simulink model "PeakDetect3"  (R2018b)
settings: Solver=FixedStepAuto  StartTime=0  StopTime=500*(15e-9)  FixedStep=15e-9  RelTol=1e-3
libraries: simulink x35, hdlsllib x34
(part 2 of 4)

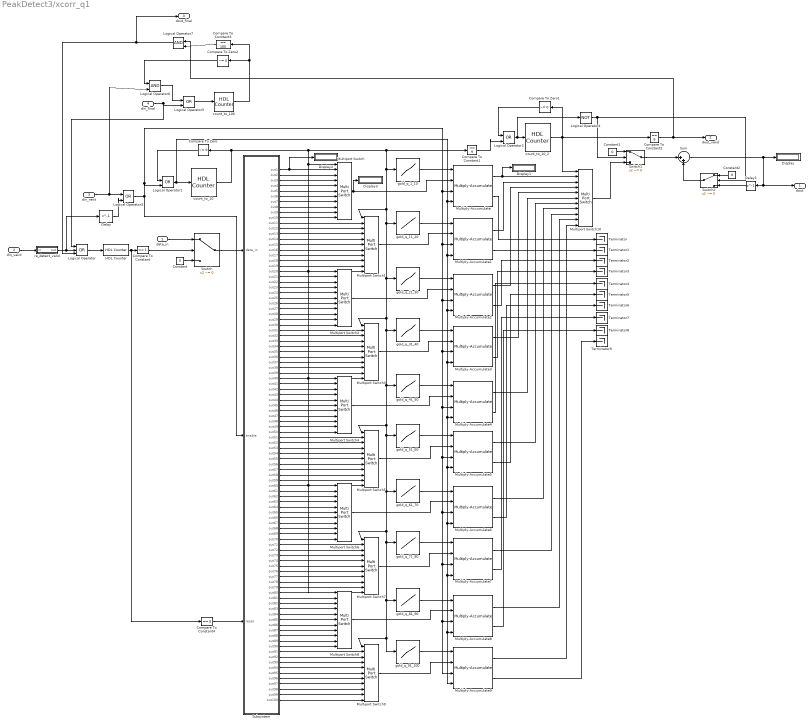
== system PeakDetect3/xcorr_q1 ==
  data_in : Inport  OutDataTypeStr=fixdt(1,16,15)
  din_valid : Inport  Port=2
  din_next : Inport  Port=3
  din_final : Inport  Port=4
  Compare To Constant : simulink/Logic and Bit Operations/Compare To Constant  relop===  const=1  OutDataTypeStr=boolean
  Compare To Constant1 : simulink/Logic and Bit Operations/Compare To Constant  relop===  const=9  OutDataTypeStr=boolean
  Compare To Constant2 : simulink/Logic and Bit Operations/Compare To Constant  relop===  const=9  OutDataTypeStr=boolean
  Compare To Constant3 : simulink/Logic and Bit Operations/Compare To Constant  relop===  const=100  OutDataTypeStr=boolean
  Compare To Constant4 : simulink/Logic and Bit Operations/Compare To Constant  relop===  const=0  OutDataTypeStr=boolean
  Compare To Zero : simulink/Logic and Bit Operations/Compare To Zero  relop=~=  OutDataTypeStr=boolean
  Compare To Zero1 : simulink/Logic and Bit Operations/Compare To Zero  relop=~=  OutDataTypeStr=boolean
  Compare To Zero2 : simulink/Logic and Bit Operations/Compare To Zero  relop=~=  OutDataTypeStr=boolean
  Constant : Constant  Value=0  OutDataTypeStr=fixdt(1,16,15)  SampleTime=-1
  Constant1 : Constant  Value=0  OutDataTypeStr=Inherit: Inherit via back propagation  SampleTime=-1
  Constant2 : Constant  Value=0  OutDataTypeStr=Inherit: Inherit via back propagation  SampleTime=-1
  Delay : Delay  DelayLength=1
  Delay1 : Delay  DelayLength=1
  Display{,1..3} (4 alike) : Display
  HDL Counter : hdlsllib/Sources/HDL Counter  CountType=Count limited  CountInit=0  CountStep=1  CountMax=2  CountFromType=Initial value  CountFrom=0  CountResetPort=off  CountLoadPort=off  CountEnbPort=on  CountDirPort=off  CountDataType=Unsigned  CountWordLen=8  CountFracLen=0  CountSampTime=1
      settings: SourceProductBaseCode=HD
  Logical Operator : Logic  Operator=OR  Inputs=3  IconShape=distinctive  AllPortsSameDT=off  OutDataTypeStr=boolean
  Logical Operator{1..3,5} (4 alike) : Logic  Operator=OR  IconShape=distinctive  AllPortsSameDT=off  OutDataTypeStr=boolean
  Logical Operator4 : Logic  Operator=NOT  IconShape=distinctive  AllPortsSameDT=off  OutDataTypeStr=boolean
  Logical Operator6 : Logic  IconShape=distinctive  AllPortsSameDT=off  OutDataTypeStr=boolean
  Logical Operator7 : Logic  IconShape=distinctive  AllPortsSameDT=off  OutDataTypeStr=boolean
  Multiply-Accumulate{,1..9} (10 alike) : hdlsllib/HDL Operations/Multiply-Accumulate  opMode=Streaming - using Start and End ports  initValueSetting=Dialog  initValue=0  initValueSetting2=Dialog  initValue2=0  initValueSetting3=Dialog  initValue3=0  num_samples=2  RndMeth2=Floor  RndMeth3=Floor  datatype2=fixdt(1,32,16)  datatype3=Inherit: Inherit via back propagation  validOut=on  endInandOut=off  startOut=off  countOut=on  dim=-1  DoSatur=off  parallel=off
      settings: SourceProductName=HDL Coder  SourceProductBaseCode=HD
  Multiport Switch{,1..9} (10 alike) : MultiPortSwitch  DataPortOrder=Zero-based contiguous  Inputs=10  zeroidx=on  OutDataTypeStr=fixdt(1,16,15)
  Multiport Switch10 : MultiPortSwitch  DataPortOrder=Zero-based contiguous  Inputs=10  zeroidx=on  OutDataTypeStr=fixdt(1,32,16)
  Subsystem : Subsystem
  Sum : Sum  Inputs=|++  OutDataTypeStr=Inherit: Inherit via back propagation
  Switch : Switch  Criteria=u2 ~= 0  OutDataTypeStr=Inherit: Inherit via back propagation
  Switch1 : Switch  Criteria=u2 ~= 0  OutDataTypeStr=Inherit: Inherit via back propagation
  Switch2 : Switch  Criteria=u2 ~= 0  OutDataTypeStr=Inherit: Inherit via back propagation
  Terminator{,1..9} (10 alike) : Terminator
  count_to_10 : hdlsllib/Sources/HDL Counter  CountType=Count limited  CountInit=0  CountStep=1  CountMax=9  CountFromType=Initial value  CountFrom=0  CountResetPort=off  CountLoadPort=off  CountEnbPort=on  CountDirPort=off  CountDataType=Unsigned  CountWordLen=4  CountFracLen=0  CountSampTime=1
      settings: SourceProductBaseCode=HD
  count_to_100 : hdlsllib/Sources/HDL Counter  CountType=Count limited  CountInit=0  CountStep=1  CountMax=100  CountFromType=Initial value  CountFrom=0  CountResetPort=off  CountLoadPort=off  CountEnbPort=on  CountDirPort=off  CountDataType=Unsigned  CountWordLen=8  CountFracLen=0  CountSampTime=1
      settings: SourceProductBaseCode=HD
  count_to_10_2 : hdlsllib/Sources/HDL Counter  CountType=Count limited  CountInit=0  CountStep=1  CountMax=9  CountFromType=Initial value  CountFrom=0  CountResetPort=off  CountLoadPort=off  CountEnbPort=on  CountDirPort=off  CountDataType=Unsigned  CountWordLen=4  CountFracLen=0  CountSampTime=1
      settings: SourceProductBaseCode=HD
  gold_q_11_20 : Lookup_n-D  NumberOfTableDimensions=1  LookupTableObject=''  BreakpointsForDimension1=uint8([0,1,2,3,4,5,6,7,8,9])  BreakpointsForDimension1FirstPoint=10  BreakpointsForDimension2FirstPoint=10  BreakpointsForDimension1Spacing=12  BreakpointsForDimension2Spacing=12  IndexSearchMethod=Evenly spaced points  Table=|  TableDataTypeStr=fixdt(1,16,15)  InterpMethod=Flat  DiagnosticForOutOfRangeInput=Error  InternalRulePriority=Speed  OutDataTypeStr=fixdt(1,16,15)  RndMeth=Simplest  InputSameDT=on
      | -1*[0.236906374990369
      | 0.265062589296935
      | 0.290853922757751
      | 0.306866645010829
      | 0.306877356493505
      | 0.282583044796408
      | 0.237895318583737
      | 0.179451570247324
      | 0.106711739895776
      | 0.0250742736874029]
  gold_q_1_10 : Lookup_n-D  NumberOfTableDimensions=1  LookupTableObject=''  BreakpointsForDimension1=uint8([0,1,2,3,4,5,6,7,8,9])  BreakpointsForDimension1FirstPoint=10  BreakpointsForDimension2FirstPoint=10  BreakpointsForDimension1Spacing=12  BreakpointsForDimension2Spacing=12  IndexSearchMethod=Evenly spaced points  Table=|  TableDataTypeStr=fixdt(1,16,15)  InterpMethod=Flat  DiagnosticForOutOfRangeInput=Error  InternalRulePriority=Speed  OutDataTypeStr=fixdt(1,16,15)  RndMeth=Simplest  InputSameDT=on
      | -1*[0.357169275362262
      | 0.373691122276015
      | 0.363136475782144
      | 0.332586509539436
      | 0.291374087870011
      | 0.249422279627694
      | 0.215579045674242
      | 0.200455944131647
      | 0.201796906991478
      | 0.213779029408702]
  gold_q_21_30 : Lookup_n-D  NumberOfTableDimensions=1  LookupTableObject=''  BreakpointsForDimension1=uint8([0,1,2,3,4,5,6,7,8,9])  BreakpointsForDimension1FirstPoint=10  BreakpointsForDimension2FirstPoint=10  BreakpointsForDimension1Spacing=12  BreakpointsForDimension2Spacing=12  IndexSearchMethod=Evenly spaced points  Table=|  TableDataTypeStr=fixdt(1,16,15)  InterpMethod=Flat  DiagnosticForOutOfRangeInput=Error  InternalRulePriority=Speed  OutDataTypeStr=fixdt(1,16,15)  RndMeth=Simplest  InputSameDT=on
      | -1*[-0.0591515848508664
      | -0.139598314313151
      | -0.210629837752387
      | -0.263713716480122
      | -0.301489962058033
      | -0.328238114626508
      | -0.340130412877520
      | -0.338689881672749
      | -0.326243180584237
      | -0.305614110780615]
  gold_q_31_40 : Lookup_n-D  NumberOfTableDimensions=1  LookupTableObject=''  BreakpointsForDimension1=uint8([0,1,2,3,4,5,6,7,8,9])  BreakpointsForDimension1FirstPoint=10  BreakpointsForDimension2FirstPoint=10  BreakpointsForDimension1Spacing=12  BreakpointsForDimension2Spacing=12  IndexSearchMethod=Evenly spaced points  Table=|  TableDataTypeStr=fixdt(1,16,15)  InterpMethod=Flat  DiagnosticForOutOfRangeInput=Error  InternalRulePriority=Speed  OutDataTypeStr=fixdt(1,16,15)  RndMeth=Simplest  InputSameDT=on
      | -1*[-0.279858098355888
      | -0.247814863771713
      | -0.225446174923891
      | -0.202743193363060
      | -0.186527042991191
      | -0.178781266249413
      | -0.180711431323688
      | -0.192575241083779
      | -0.213551675353351
      | -0.245925394077466]
  gold_q_41_50 : Lookup_n-D  NumberOfTableDimensions=1  LookupTableObject=''  BreakpointsForDimension1=uint8([0,1,2,3,4,5,6,7,8,9])  BreakpointsForDimension1FirstPoint=10  BreakpointsForDimension2FirstPoint=10  BreakpointsForDimension1Spacing=12  BreakpointsForDimension2Spacing=12  IndexSearchMethod=Evenly spaced points  Table=|  TableDataTypeStr=fixdt(1,16,15)  InterpMethod=Flat  DiagnosticForOutOfRangeInput=Error  InternalRulePriority=Speed  OutDataTypeStr=fixdt(1,16,15)  RndMeth=Simplest  InputSameDT=on
      | -1*[-0.273649789754997
      | -0.305507933389466
      | -0.332526349511340
      | -0.349961882407133
      | -0.353614169955030
      | -0.340366684130075
      | -0.308641627170326
      | -0.254460428744123
      | -0.185247665828561
      | -0.110080691949015]
  gold_q_51_60 : Lookup_n-D  NumberOfTableDimensions=1  LookupTableObject=''  BreakpointsForDimension1=uint8([0,1,2,3,4,5,6,7,8,9])  BreakpointsForDimension1FirstPoint=10  BreakpointsForDimension2FirstPoint=10  BreakpointsForDimension1Spacing=12  BreakpointsForDimension2Spacing=12  IndexSearchMethod=Evenly spaced points  Table=|  TableDataTypeStr=fixdt(1,16,15)  InterpMethod=Flat  DiagnosticForOutOfRangeInput=Error  InternalRulePriority=Speed  OutDataTypeStr=fixdt(1,16,15)  RndMeth=Simplest  InputSameDT=on
      | -1*[-0.0297558495000079
      | 0.0499350486257353
      | 0.122950591883728
      | 0.183532283875116
      | 0.226715241693549
      | 0.244522518247979
      | 0.247772413924009
      | 0.223279362418140
      | 0.176793915855740
      | 0.111355596734925]
  gold_q_61_70 : Lookup_n-D  NumberOfTableDimensions=1  LookupTableObject=''  BreakpointsForDimension1=uint8([0,1,2,3,4,5,6,7,8,9])  BreakpointsForDimension1FirstPoint=10  BreakpointsForDimension2FirstPoint=10  BreakpointsForDimension1Spacing=12  BreakpointsForDimension2Spacing=12  IndexSearchMethod=Evenly spaced points  Table=|  TableDataTypeStr=fixdt(1,16,15)  InterpMethod=Flat  DiagnosticForOutOfRangeInput=Error  InternalRulePriority=Speed  OutDataTypeStr=fixdt(1,16,15)  RndMeth=Simplest  InputSameDT=on
      | -1*[0.0312880626224120
      | -0.0580988665112754
      | -0.150830519884918
      | -0.236354458852815
      | -0.321361371110983
      | -0.387151947785857
      | -0.432910784333285
      | -0.454553321854592
      | -0.449340647995131
      | -0.416266380216616]
  gold_q_71_80 : Lookup_n-D  NumberOfTableDimensions=1  LookupTableObject=''  BreakpointsForDimension1=uint8([0,1,2,3,4,5,6,7,8,9])  BreakpointsForDimension1FirstPoint=10  BreakpointsForDimension2FirstPoint=10  BreakpointsForDimension1Spacing=12  BreakpointsForDimension2Spacing=12  IndexSearchMethod=Evenly spaced points  Table=|  TableDataTypeStr=fixdt(1,16,15)  InterpMethod=Flat  DiagnosticForOutOfRangeInput=Error  InternalRulePriority=Speed  OutDataTypeStr=fixdt(1,16,15)  RndMeth=Simplest  InputSameDT=on
      | -1*[-0.356405677154333
      | -0.268905527196357
      | -0.172503144328213
      | -0.0623088722264564
      | 0.0478292512438748
      | 0.147701871156711
      | 0.227579808283800
      | 0.279365016179912
      | 0.297653875710056
      | 0.276310228166542]
  gold_q_81_90 : Lookup_n-D  NumberOfTableDimensions=1  LookupTableObject=''  BreakpointsForDimension1=uint8([0,1,2,3,4,5,6,7,8,9])  BreakpointsForDimension1FirstPoint=10  BreakpointsForDimension2FirstPoint=10  BreakpointsForDimension1Spacing=12  BreakpointsForDimension2Spacing=12  IndexSearchMethod=Evenly spaced points  Table=|  TableDataTypeStr=fixdt(1,16,15)  InterpMethod=Flat  DiagnosticForOutOfRangeInput=Error  InternalRulePriority=Speed  OutDataTypeStr=fixdt(1,16,15)  RndMeth=Simplest  InputSameDT=on
      | -1*[0.222595237130309
      | 0.147485843722747
      | 0.0555170073150737
      | -0.0424496465550990
      | -0.134707118174198
      | -0.210100315272752
      | -0.259403813850479
      | -0.272248751146779
      | -0.259403813850479
      | -0.210100315272752]
  gold_q_91_100 : Lookup_n-D  NumberOfTableDimensions=1  LookupTableObject=''  BreakpointsForDimension1=uint8([0,1,2,3,4,5,6,7,8,9])  BreakpointsForDimension1FirstPoint=10  BreakpointsForDimension2FirstPoint=10  BreakpointsForDimension1Spacing=12  BreakpointsForDimension2Spacing=12  IndexSearchMethod=Evenly spaced points  Table=|  TableDataTypeStr=fixdt(1,16,15)  InterpMethod=Flat  DiagnosticForOutOfRangeInput=Error  InternalRulePriority=Speed  OutDataTypeStr=fixdt(1,16,15)  RndMeth=Simplest  InputSameDT=on
      | -1*[-0.134707118174198
      | -0.0424496465550989
      | 0.0555170073150737
      | 0.147485843722747
      | 0.222595237130309
      | 0.267820298855522
      | 0.290378842162360
      | 0.275261187855880
      | 0.228204197191429
      | 0.153805243290024]
  re_detect_valid : Subsystem
  dout : Outport  OutDataTypeStr=fixdt(1,32,16)
  dout_valid : Outport  Port=2
  dout_final : Outport  Port=3
  wires:
  Subsystem/63(out63) -> Multiport Switch6/4
  Subsystem/83(out83) -> Multiport Switch8/4
  Subsystem/87(out87) -> Multiport Switch8/8
  Subsystem/57(out57) -> Multiport Switch5/8
  count_to_10/1 -> Compare To Zero/1, Multiport Switch8/1, Multiport Switch6/1, Multiport Switch4/1, Multiport Switch2/1, Multiport Switch/1, gold_q_11_20/1, gold_q_21_30/1, gold_q_31_40/1, gold_q_41_50/1, gold_q_51_60/1, gold_q_61_70/1, gold_q_71_80/1, gold_q_81_90/1, gold_q_91_100/1, Multiport Switch9/1, Multiport Switch7/1, Multiport Switch5/1, Multiport Switch3/1, Multiport Switch1/1, gold_q_1_10/1, Compare To Constant1/1
  Subsystem/97(out97) -> Multiport Switch9/8
  Multiply-Accumulate4/1 -> Multiport Switch10/6
  Subsystem/65(out65) -> Multiport Switch6/6
  Subsystem/99(out99) -> Multiport Switch9/10
  Subsystem/73(out73) -> Multiport Switch7/4
  Subsystem/49(out49) -> Multiport Switch4/10
  Multiply-Accumulate/2 -> Terminator/1
  din_final/1 -> Logical Operator/1, Logical Operator5/2
  count_to_10_2/1 -> Compare To Constant2/1, Multiport Switch10/1, Compare To Zero1/1
  Multiport Switch8/1 -> Multiply-Accumulate8/2
  Compare To Constant2/1 -> dout_valid/1, Logical Operator7/1
  Subsystem/61(out61) -> Multiport Switch6/2
  Subsystem/28(out28) -> Multiport Switch2/9
  Subsystem/1(out1) -> Display2/1, Multiport Switch/2
  Multiply-Accumulate6/1 -> Multiport Switch10/8
  Subsystem/100(out100) -> Multiport Switch9/11
  Logical Operator/1 -> HDL Counter/1
  din_valid/1 -> re_detect_valid/1(in)
  Subsystem/68(out68) -> Multiport Switch6/9
  Subsystem/56(out56) -> Multiport Switch5/7
  Subsystem/13(out13) -> Multiport Switch1/4
  Subsystem/67(out67) -> Multiport Switch6/8
  Subsystem/66(out66) -> Multiport Switch6/7
  Logical Operator2/1 -> Logical Operator4/1, count_to_10_2/1
  Constant/1 -> Switch/3
  Compare To Zero/1 -> Logical Operator1/1
  Subsystem/89(out89) -> Multiport Switch8/10
  Multiport Switch5/1 -> Multiply-Accumulate5/2
  Subsystem/29(out29) -> Multiport Switch2/10
  Compare To Constant/1 -> Switch/2
  gold_q_91_100/1 -> Multiply-Accumulate9/1
  Subsystem/52(out52) -> Multiport Switch5/3
  re_detect_valid/1(out) -> Delay/1, Logical Operator/2
  Logical Operator1/1 -> count_to_10/1, Multiply-Accumulate2/4, Multiply-Accumulate9/4, Multiply-Accumulate8/4, Multiply-Accumulate7/4, Multiply-Accumulate6/4, Multiply-Accumulate5/4, Multiply-Accumulate4/4, Multiply-Accumulate3/4, Multiply-Accumulate1/4, Multiply-Accumulate/4
  Subsystem/76(out76) -> Multiport Switch7/7
  Sum/1 -> dout/1, Delay1/1, Display/1
  Logical Operator3/1 -> Subsystem/2(enable), Multiply-Accumulate9/3, Multiply-Accumulate8/3, Multiply-Accumulate7/3, Multiply-Accumulate6/3, Multiply-Accumulate5/3, Multiply-Accumulate4/3, Multiply-Accumulate3/3, Multiply-Accumulate2/3, Multiply-Accumulate1/3, Multiply-Accumulate/3, Logical Operator1/2
  Subsystem/2(out2) -> Multiport Switch/3
  Subsystem/88(out88) -> Multiport Switch8/9
  Subsystem/64(out64) -> Multiport Switch6/5
  Subsystem/41(out41) -> Multiport Switch4/2
  Multiply-Accumulate9/2 -> Terminator9/1
  din_next/1 -> Logical Operator6/2, Logical Operator3/1
  Subsystem/11(out11) -> Multiport Switch1/2
  Subsystem/96(out96) -> Multiport Switch9/7
  Switch1/1 -> Sum/1
  Subsystem/80(out80) -> Multiport Switch7/11
  Subsystem/54(out54) -> Multiport Switch5/5
  Subsystem/82(out82) -> Multiport Switch8/3
  Multiply-Accumulate4/2 -> Terminator4/1
  Subsystem/6(out6) -> Multiport Switch/7
  Subsystem/45(out45) -> Multiport Switch4/6
  Multiport Switch4/1 -> Multiply-Accumulate4/2
  Logical Operator4/1 -> Switch1/2, Switch2/2
  Subsystem/58(out58) -> Multiport Switch5/9
  Subsystem/81(out81) -> Multiport Switch8/2
  Subsystem/44(out44) -> Multiport Switch4/5
  Subsystem/86(out86) -> Multiport Switch8/7
  Subsystem/85(out85) -> Multiport Switch8/6
  Logical Operator5/1 -> count_to_100/1
  Multiport Switch/1 -> Multiply-Accumulate/2, Display3/1
  Subsystem/27(out27) -> Multiport Switch2/8
  gold_q_31_40/1 -> Multiply-Accumulate3/1
  Subsystem/93(out93) -> Multiport Switch9/4
  Compare To Zero1/1 -> Logical Operator2/1
  Subsystem/39(out39) -> Multiport Switch3/10
  Subsystem/84(out84) -> Multiport Switch8/5
  Subsystem/70(out70) -> Multiport Switch6/11
  Subsystem/77(out77) -> Multiport Switch7/8
  Subsystem/62(out62) -> Multiport Switch6/3
  Subsystem/95(out95) -> Multiport Switch9/6
  gold_q_1_10/1 -> Multiply-Accumulate/1
  Compare To Zero2/1 -> Logical Operator6/1
  Multiply-Accumulate1/1 -> Multiport Switch10/3
  Subsystem/47(out47) -> Multiport Switch4/8
  Multiply-Accumulate3/2 -> Terminator3/1
  Subsystem/22(out22) -> Multiport Switch2/3
  Subsystem/92(out92) -> Multiport Switch9/3
  count_to_100/1 -> Compare To Constant3/1, Compare To Zero2/1
  Multiport Switch3/1 -> Multiply-Accumulate3/2
  Subsystem/59(out59) -> Multiport Switch5/10
  Subsystem/9(out9) -> Multiport Switch/10
  Subsystem/5(out5) -> Multiport Switch/6
  gold_q_11_20/1 -> Multiply-Accumulate1/1
  data_in/1 -> Switch/1
  Subsystem/90(out90) -> Multiport Switch8/11
  Subsystem/10(out10) -> Multiport Switch/11
  Subsystem/75(out75) -> Multiport Switch7/6
  Subsystem/18(out18) -> Multiport Switch1/9
  Subsystem/12(out12) -> Multiport Switch1/3
  Subsystem/25(out25) -> Multiport Switch2/6
  Subsystem/43(out43) -> Multiport Switch4/4
  Subsystem/72(out72) -> Multiport Switch7/3
  Subsystem/30(out30) -> Multiport Switch2/11
  Subsystem/8(out8) -> Multiport Switch/9
  Subsystem/60(out60) -> Multiport Switch5/11
  HDL Counter/1 -> Compare To Constant4/1, Compare To Constant/1
  Multiply-Accumulate8/2 -> Terminator8/1
  Subsystem/17(out17) -> Multiport Switch1/8
  Multiply-Accumulate9/1 -> Multiport Switch10/11
  Subsystem/26(out26) -> Multiport Switch2/7
  Subsystem/35(out35) -> Multiport Switch3/6
  Subsystem/24(out24) -> Multiport Switch2/5
  Subsystem/20(out20) -> Multiport Switch1/11
  Subsystem/71(out71) -> Multiport Switch7/2
  Subsystem/78(out78) -> Multiport Switch7/9
  Multiport Switch9/1 -> Multiply-Accumulate9/2
  Subsystem/7(out7) -> Multiport Switch/8
  Subsystem/3(out3) -> Multiport Switch/4
  Subsystem/79(out79) -> Multiport Switch7/10
  Multiport Switch10/1 -> Switch1/3
  Subsystem/15(out15) -> Multiport Switch1/6
  Subsystem/14(out14) -> Multiport Switch1/5
  Multiply-Accumulate/1 -> Display1/1, Multiport Switch10/2
  Subsystem/42(out42) -> Multiport Switch4/3
  Subsystem/16(out16) -> Multiport Switch1/7
  Logical Operator6/1 -> Logical Operator5/1
  Logical Operator7/1 -> dout_final/1, Logical Operator/3
  Subsystem/53(out53) -> Multiport Switch5/4
  Subsystem/37(out37) -> Multiport Switch3/8
  Subsystem/55(out55) -> Multiport Switch5/6
  Subsystem/48(out48) -> Multiport Switch4/9
  Subsystem/4(out4) -> Multiport Switch/5
  Subsystem/50(out50) -> Multiport Switch4/11
  Subsystem/40(out40) -> Multiport Switch3/11
  Switch/1 -> Subsystem/1(data_in)
  Subsystem/19(out19) -> Multiport Switch1/10
  Subsystem/38(out38) -> Multiport Switch3/9
  Subsystem/33(out33) -> Multiport Switch3/4
  Subsystem/46(out46) -> Multiport Switch4/7
  Subsystem/31(out31) -> Multiport Switch3/2
  Subsystem/69(out69) -> Multiport Switch6/10
  Subsystem/94(out94) -> Multiport Switch9/5
  gold_q_71_80/1 -> Multiply-Accumulate7/1
  Subsystem/32(out32) -> Multiport Switch3/3
  Multiply-Accumulate3/1 -> Multiport Switch10/5
  Subsystem/23(out23) -> Multiport Switch2/4
  Multiply-Accumulate2/1 -> Multiport Switch10/4
  Multiport Switch6/1 -> Multiply-Accumulate6/2
  Constant1/1 -> Switch1/1
  Multiply-Accumulate6/2 -> Terminator6/1
  Compare To Constant1/1 -> Logical Operator2/2
  Constant2/1 -> Switch2/1
  Compare To Constant3/1 -> Logical Operator7/2
  gold_q_41_50/1 -> Multiply-Accumulate4/1
  gold_q_21_30/1 -> Multiply-Accumulate2/1
  Multiport Switch2/1 -> Multiply-Accumulate2/2
  Subsystem/21(out21) -> Multiport Switch2/2
  gold_q_61_70/1 -> Multiply-Accumulate6/1
  gold_q_51_60/1 -> Multiply-Accumulate5/1
  Multiply-Accumulate7/1 -> Multiport Switch10/9
  Multiport Switch7/1 -> Multiply-Accumulate7/2
  gold_q_81_90/1 -> Multiply-Accumulate8/1
  Multiport Switch1/1 -> Multiply-Accumulate1/2
  Subsystem/91(out91) -> Multiport Switch9/2
  Multiply-Accumulate5/1 -> Multiport Switch10/7
  Multiply-Accumulate8/1 -> Multiport Switch10/10
  Delay/1 -> Logical Operator3/2
  Delay1/1 -> Switch2/3
  Switch2/1 -> Sum/2
  Subsystem/51(out51) -> Multiport Switch5/2
  Subsystem/36(out36) -> Multiport Switch3/7
  Subsystem/34(out34) -> Multiport Switch3/5
  Compare To Constant4/1 -> Subsystem/3(reset)
  Subsystem/98(out98) -> Multiport Switch9/9
  Multiply-Accumulate5/2 -> Terminator5/1
  Subsystem/74(out74) -> Multiport Switch7/5
  Multiply-Accumulate7/2 -> Terminator7/1
  Multiply-Accumulate1/2 -> Terminator1/1
  Multiply-Accumulate2/2 -> Terminator2/1

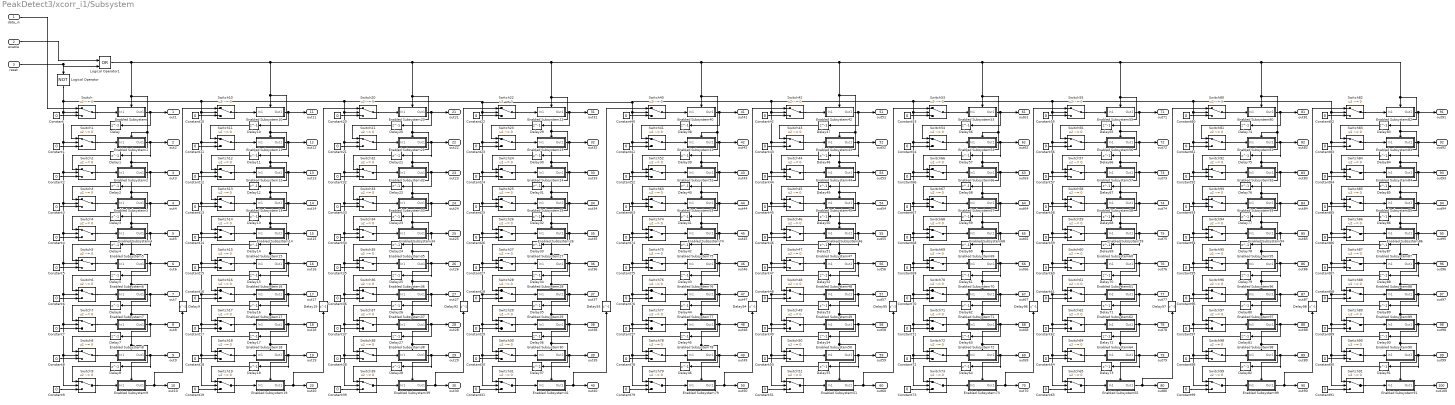
== system PeakDetect3/xcorr_i1/Subsystem ==
  data_in : Inport  OutDataTypeStr=fixdt(1,16,15)
  enable : Inport  Port=2
  reset : Inport  Port=3
  Constant{,1..99} (100 alike) : Constant  Value=0  OutDataTypeStr=Inherit: Inherit via back propagation  SampleTime=-1
  Delay{,1..98} (99 alike) : Delay  DelayLength=1
  Enabled Subsystem : Subsystem  TreatAsAtomicUnit=on
  Enabled Subsystem1 : Subsystem  TreatAsAtomicUnit=on
  Enabled Subsystem10 : Subsystem  TreatAsAtomicUnit=on
  Enabled Subsystem11 : Subsystem  TreatAsAtomicUnit=on
  Enabled Subsystem12 : Subsystem  TreatAsAtomicUnit=on
  Enabled Subsystem13 : Subsystem  TreatAsAtomicUnit=on
  Enabled Subsystem14 : Subsystem  TreatAsAtomicUnit=on
  Enabled Subsystem15 : Subsystem  TreatAsAtomicUnit=on
  Enabled Subsystem16 : Subsystem  TreatAsAtomicUnit=on
  Enabled Subsystem17 : Subsystem  TreatAsAtomicUnit=on
  Enabled Subsystem18 : Subsystem  TreatAsAtomicUnit=on
  Enabled Subsystem19 : Subsystem  TreatAsAtomicUnit=on
  Enabled Subsystem2 : Subsystem  TreatAsAtomicUnit=on
  Enabled Subsystem20 : Subsystem  TreatAsAtomicUnit=on
  Enabled Subsystem21 : Subsystem  TreatAsAtomicUnit=on
  Enabled Subsystem22 : Subsystem  TreatAsAtomicUnit=on
  Enabled Subsystem23 : Subsystem  TreatAsAtomicUnit=on
  Enabled Subsystem24 : Subsystem  TreatAsAtomicUnit=on
  Enabled Subsystem25 : Subsystem  TreatAsAtomicUnit=on
  Enabled Subsystem26 : Subsystem  TreatAsAtomicUnit=on
  Enabled Subsystem27 : Subsystem  TreatAsAtomicUnit=on
  Enabled Subsystem28 : Subsystem  TreatAsAtomicUnit=on
  Enabled Subsystem29 : Subsystem  TreatAsAtomicUnit=on
  Enabled Subsystem3 : Subsystem  TreatAsAtomicUnit=on
  Enabled Subsystem30 : Subsystem  TreatAsAtomicUnit=on
  Enabled Subsystem31 : Subsystem  TreatAsAtomicUnit=on
  Enabled Subsystem32 : Subsystem  TreatAsAtomicUnit=on
  Enabled Subsystem33 : Subsystem  TreatAsAtomicUnit=on
  Enabled Subsystem34 : Subsystem  TreatAsAtomicUnit=on
  Enabled Subsystem35 : Subsystem  TreatAsAtomicUnit=on
  Enabled Subsystem36 : Subsystem  TreatAsAtomicUnit=on
  Enabled Subsystem37 : Subsystem  TreatAsAtomicUnit=on
  Enabled Subsystem38 : Subsystem  TreatAsAtomicUnit=on
  Enabled Subsystem39 : Subsystem  TreatAsAtomicUnit=on
  Enabled Subsystem4 : Subsystem  TreatAsAtomicUnit=on
  Enabled Subsystem40 : Subsystem  TreatAsAtomicUnit=on
  Enabled Subsystem41 : Subsystem  TreatAsAtomicUnit=on
  Enabled Subsystem42 : Subsystem  TreatAsAtomicUnit=on
  Enabled Subsystem43 : Subsystem  TreatAsAtomicUnit=on
  Enabled Subsystem44 : Subsystem  TreatAsAtomicUnit=on
  Enabled Subsystem45 : Subsystem  TreatAsAtomicUnit=on
  Enabled Subsystem46 : Subsystem  TreatAsAtomicUnit=on
  Enabled Subsystem47 : Subsystem  TreatAsAtomicUnit=on
  Enabled Subsystem48 : Subsystem  TreatAsAtomicUnit=on
  Enabled Subsystem49 : Subsystem  TreatAsAtomicUnit=on
  Enabled Subsystem5 : Subsystem  TreatAsAtomicUnit=on
  Enabled Subsystem50 : Subsystem  TreatAsAtomicUnit=on
  Enabled Subsystem51 : Subsystem  TreatAsAtomicUnit=on
  Enabled Subsystem52 : Subsystem  TreatAsAtomicUnit=on
  Enabled Subsystem53 : Subsystem  TreatAsAtomicUnit=on
  Enabled Subsystem54 : Subsystem  TreatAsAtomicUnit=on
  Enabled Subsystem55 : Subsystem  TreatAsAtomicUnit=on
  Enabled Subsystem56 : Subsystem  TreatAsAtomicUnit=on
  Enabled Subsystem57 : Subsystem  TreatAsAtomicUnit=on
  Enabled Subsystem58 : Subsystem  TreatAsAtomicUnit=on
  Enabled Subsystem59 : Subsystem  TreatAsAtomicUnit=on
  Enabled Subsystem6 : Subsystem  TreatAsAtomicUnit=on
  Enabled Subsystem60 : Subsystem  TreatAsAtomicUnit=on
  Enabled Subsystem61 : Subsystem  TreatAsAtomicUnit=on
  Enabled Subsystem62 : Subsystem  TreatAsAtomicUnit=on
  Enabled Subsystem63 : Subsystem  TreatAsAtomicUnit=on
  Enabled Subsystem64 : Subsystem  TreatAsAtomicUnit=on
  Enabled Subsystem65 : Subsystem  TreatAsAtomicUnit=on
  Enabled Subsystem66 : Subsystem  TreatAsAtomicUnit=on
  Enabled Subsystem67 : Subsystem  TreatAsAtomicUnit=on
  Enabled Subsystem68 : Subsystem  TreatAsAtomicUnit=on
  Enabled Subsystem69 : Subsystem  TreatAsAtomicUnit=on
  Enabled Subsystem7 : Subsystem  TreatAsAtomicUnit=on
  Enabled Subsystem70 : Subsystem  TreatAsAtomicUnit=on
  Enabled Subsystem71 : Subsystem  TreatAsAtomicUnit=on
  Enabled Subsystem72 : Subsystem  TreatAsAtomicUnit=on
  Enabled Subsystem73 : Subsystem  TreatAsAtomicUnit=on
  Enabled Subsystem74 : Subsystem  TreatAsAtomicUnit=on
  Enabled Subsystem75 : Subsystem  TreatAsAtomicUnit=on
  Enabled Subsystem76 : Subsystem  TreatAsAtomicUnit=on
  Enabled Subsystem77 : Subsystem  TreatAsAtomicUnit=on
  Enabled Subsystem78 : Subsystem  TreatAsAtomicUnit=on
  Enabled Subsystem79 : Subsystem  TreatAsAtomicUnit=on
  Enabled Subsystem8 : Subsystem  TreatAsAtomicUnit=on
  Enabled Subsystem80 : Subsystem  TreatAsAtomicUnit=on
  Enabled Subsystem81 : Subsystem  TreatAsAtomicUnit=on
  Enabled Subsystem82 : Subsystem  TreatAsAtomicUnit=on
  Enabled Subsystem83 : Subsystem  TreatAsAtomicUnit=on
  Enabled Subsystem84 : Subsystem  TreatAsAtomicUnit=on
  Enabled Subsystem85 : Subsystem  TreatAsAtomicUnit=on
  Enabled Subsystem86 : Subsystem  TreatAsAtomicUnit=on
  Enabled Subsystem87 : Subsystem  TreatAsAtomicUnit=on
  Enabled Subsystem88 : Subsystem  TreatAsAtomicUnit=on
  Enabled Subsystem89 : Subsystem  TreatAsAtomicUnit=on
  Enabled Subsystem9 : Subsystem  TreatAsAtomicUnit=on
  Enabled Subsystem90 : Subsystem  TreatAsAtomicUnit=on
  Enabled Subsystem91 : Subsystem  TreatAsAtomicUnit=on
  Enabled Subsystem92 : Subsystem  TreatAsAtomicUnit=on
  Enabled Subsystem93 : Subsystem  TreatAsAtomicUnit=on
  Enabled Subsystem94 : Subsystem  TreatAsAtomicUnit=on
  Enabled Subsystem95 : Subsystem  TreatAsAtomicUnit=on
  Enabled Subsystem96 : Subsystem  TreatAsAtomicUnit=on
  Enabled Subsystem97 : Subsystem  TreatAsAtomicUnit=on
  Enabled Subsystem98 : Subsystem  TreatAsAtomicUnit=on
  Enabled Subsystem99 : Subsystem  TreatAsAtomicUnit=on
  Logical Operator : Logic  Operator=NOT  IconShape=distinctive  AllPortsSameDT=off  OutDataTypeStr=boolean
  Logical Operator1 : Logic  Operator=OR  IconShape=distinctive  AllPortsSameDT=off  OutDataTypeStr=boolean
  Switch{,1..99} (100 alike) : Switch  Criteria=u2 ~= 0  OutDataTypeStr=Inherit: Inherit via back propagation
  out1 : Outport
  out2 : Outport  Port=2
  out3 : Outport  Port=3
  out4 : Outport  Port=4
  out5 : Outport  Port=5
  out6 : Outport  Port=6
  out7 : Outport  Port=7
  out8 : Outport  Port=8
  out9 : Outport  Port=9
  out10 : Outport  Port=10
  out11 : Outport  Port=11
  out12 : Outport  Port=12
  out13 : Outport  Port=13
  out14 : Outport  Port=14
  out15 : Outport  Port=15
  out16 : Outport  Port=16
  out17 : Outport  Port=17
  out18 : Outport  Port=18
  out19 : Outport  Port=19
  out20 : Outport  Port=20
  out21 : Outport  Port=21
  out22 : Outport  Port=22
  out23 : Outport  Port=23
  out24 : Outport  Port=24
  out25 : Outport  Port=25
  out26 : Outport  Port=26
  out27 : Outport  Port=27
  out28 : Outport  Port=28
  out29 : Outport  Port=29
  out30 : Outport  Port=30
  out31 : Outport  Port=31
  out32 : Outport  Port=32
  out33 : Outport  Port=33
  out34 : Outport  Port=34
  out35 : Outport  Port=35
  out36 : Outport  Port=36
  out37 : Outport  Port=37
  out38 : Outport  Port=38
  out39 : Outport  Port=39
  out40 : Outport  Port=40
  out41 : Outport  Port=41
  out42 : Outport  Port=42
  out43 : Outport  Port=43
  out44 : Outport  Port=44
  out45 : Outport  Port=45
  out46 : Outport  Port=46
  out47 : Outport  Port=47
  out48 : Outport  Port=48
  out49 : Outport  Port=49
  out50 : Outport  Port=50
  out51 : Outport  Port=51
  out52 : Outport  Port=52
  out53 : Outport  Port=53
  out54 : Outport  Port=54
  out55 : Outport  Port=55
  out56 : Outport  Port=56
  out57 : Outport  Port=57
  out58 : Outport  Port=58
  out59 : Outport  Port=59
  out60 : Outport  Port=60
  out61 : Outport  Port=61
  out62 : Outport  Port=62
  out63 : Outport  Port=63
  out64 : Outport  Port=64
  out65 : Outport  Port=65
  out66 : Outport  Port=66
  out67 : Outport  Port=67
  out68 : Outport  Port=68
  out69 : Outport  Port=69
  out70 : Outport  Port=70
  out71 : Outport  Port=71
  out72 : Outport  Port=72
  out73 : Outport  Port=73
  out74 : Outport  Port=74
  out75 : Outport  Port=75
  out76 : Outport  Port=76
  out77 : Outport  Port=77
  out78 : Outport  Port=78
  out79 : Outport  Port=79
  out80 : Outport  Port=80
  out81 : Outport  Port=81
  out82 : Outport  Port=82
  out83 : Outport  Port=83
  out84 : Outport  Port=84
  out85 : Outport  Port=85
  out86 : Outport  Port=86
  out87 : Outport  Port=87
  out88 : Outport  Port=88
  out89 : Outport  Port=89
  out90 : Outport  Port=90
  out91 : Outport  Port=91
  out92 : Outport  Port=92
  out93 : Outport  Port=93
  out94 : Outport  Port=94
  out95 : Outport  Port=95
  out96 : Outport  Port=96
  out97 : Outport  Port=97
  out98 : Outport  Port=98
  out99 : Outport  Port=99
  out100 : Outport  Port=100
  wires:
  Delay81/1 -> Switch98/1
  Delay36/1 -> Switch30/1
  Constant37/1 -> Switch37/3
  Switch72/1 -> Enabled Subsystem72/1(In1)
  Switch33/1 -> Enabled Subsystem33/1(In1)
  Delay65/1 -> Switch56/1
  Constant39/1 -> Switch39/3
  Switch76/1 -> Enabled Subsystem76/1(In1)
  Constant59/1 -> Switch59/3
  Constant70/1 -> Switch70/3
  Constant12/1 -> Switch12/3
  Constant58/1 -> Switch58/3
  Delay52/1 -> Switch48/1
  Switch58/1 -> Enabled Subsystem58/1(In1)
  Constant55/1 -> Switch55/3
  Switch29/1 -> Enabled Subsystem29/1(In1)
  Switch37/1 -> Enabled Subsystem37/1(In1)
  Constant99/1 -> Switch99/3
  Constant22/1 -> Switch22/3
  Constant34/1 -> Switch34/3
  Switch38/1 -> Enabled Subsystem38/1(In1)
  Delay/1 -> Switch1/1
  Switch23/1 -> Enabled Subsystem23/1(In1)
  Delay25/1 -> Switch36/1
  Delay22/1 -> Switch33/1
  Delay50/1 -> Switch46/1
  Constant53/1 -> Switch53/3
  Enabled Subsystem97/1(Out1) -> out88/1, Delay81/1
  Switch45/1 -> Enabled Subsystem45/1(In1)
  Switch6/1 -> Enabled Subsystem6/1(In1)
  Delay92/1 -> Switch22/1
  Switch55/1 -> Enabled Subsystem55/1(In1)
  Constant38/1 -> Switch38/3
  Delay58/1 -> Switch67/1
  Enabled Subsystem76/1(Out1) -> out47/1, Delay44/1
  Constant54/1 -> Switch54/3
  Constant31/1 -> Switch31/3
  Enabled Subsystem39/1(Out1) -> out30/1, Delay92/1
  Delay94/1 -> Switch42/1
  Switch90/1 -> Enabled Subsystem90/1(In1)
  Delay8/1 -> Switch9/1
  Constant50/1 -> Switch50/3
  Enabled Subsystem55/1(Out1) -> out71/1, Delay65/1
  Delay72/1 -> Switch64/1
  Constant76/1 -> Switch76/3
  Switch73/1 -> Enabled Subsystem73/1(In1)
  Constant41/1 -> Switch41/3
  Constant97/1 -> Switch97/3
  Switch44/1 -> Enabled Subsystem44/1(In1)
  Switch77/1 -> Enabled Subsystem77/1(In1)
  Constant47/1 -> Switch47/3
  Constant62/1 -> Switch62/3
  Switch3/1 -> Enabled Subsystem3/1(In1)
  Constant71/1 -> Switch71/3
  Delay37/1 -> Switch31/1
  Constant75/1 -> Switch75/3
  Constant93/1 -> Switch93/3
  Switch2/1 -> Enabled Subsystem2/1(In1)
  Constant29/1 -> Switch29/3
  Enabled Subsystem72/1(Out1) -> out69/1, Delay64/1
  Delay24/1 -> Switch35/1
  Constant56/1 -> Switch56/3
  Switch8/1 -> Enabled Subsystem8/1(In1)
  Switch31/1 -> Enabled Subsystem31/1(In1)
  Delay89/1 -> Switch89/1
  Delay27/1 -> Switch38/1
  Constant2/1 -> Switch2/3
  Switch13/1 -> Enabled Subsystem13/1(In1)
  Constant/1 -> Switch/3
  Delay64/1 -> Switch73/1
  Constant81/1 -> Switch81/3
  Constant40/1 -> Switch40/3
  Switch52/1 -> Enabled Subsystem52/1(In1)
  Switch14/1 -> Enabled Subsystem14/1(In1)
  Enabled Subsystem17/1(Out1) -> out18/1, Delay17/1
  Constant49/1 -> Switch49/3
  Switch70/1 -> Enabled Subsystem70/1(In1)
  Constant64/1 -> Switch64/3
  Switch82/1 -> Enabled Subsystem82/1(In1)
  Delay98/1 -> Switch82/1
  Enabled Subsystem77/1(Out1) -> out48/1, Delay45/1
  Enabled Subsystem59/1(Out1) -> out75/1, Delay69/1
  Constant68/1 -> Switch68/3
  Enabled Subsystem1/1(Out1) -> out2/1, Delay1/1
  Constant92/1 -> Switch92/3
  Enabled Subsystem52/1(Out1) -> out43/1, Delay40/1
  Enabled Subsystem36/1(Out1) -> out27/1, Delay26/1
  Delay86/1 -> Switch86/1
  Constant83/1 -> Switch83/3
  Switch83/1 -> Enabled Subsystem83/1(In1)
  Enabled Subsystem63/1(Out1) -> out44/1, Delay41/1
  Switch15/1 -> Enabled Subsystem15/1(In1)
  Constant46/1 -> Switch46/3
  Delay39/1 -> Switch52/1
  Delay31/1 -> Switch25/1
  Constant6/1 -> Switch6/3
  Switch26/1 -> Enabled Subsystem26/1(In1)
  Delay29/1 -> Switch23/1
  Constant28/1 -> Switch28/3
  Constant11/1 -> Switch11/3
  Constant9/1 -> Switch9/3
  Enabled Subsystem5/1(Out1) -> out6/1, Delay5/1
  Delay48/1 -> Switch44/1
  Switch4/1 -> Enabled Subsystem4/1(In1)
  Delay77/1 -> Switch94/1
  Constant24/1 -> Switch24/3
  Switch17/1 -> Enabled Subsystem17/1(In1)
  Switch32/1 -> Enabled Subsystem32/1(In1)
  Enabled Subsystem49/1(Out1) -> out58/1, Delay54/1
  Constant73/1 -> Switch73/3
  Switch34/1 -> Enabled Subsystem34/1(In1)
  Delay76/1 -> Switch93/1
  Enabled Subsystem48/1(Out1) -> out57/1, Delay53/1
  Switch74/1 -> Enabled Subsystem74/1(In1)
  Enabled Subsystem53/1(Out1) -> out61/1, Delay56/1
  Enabled Subsystem44/1(Out1) -> out53/1, Delay49/1
  Delay90/1 -> Switch90/1
  Constant61/1 -> Switch61/3
  Switch63/1 -> Enabled Subsystem63/1(In1)
  Switch89/1 -> Enabled Subsystem89/1(In1)
  Switch94/1 -> Enabled Subsystem94/1(In1)
  Delay67/1 -> Switch58/1
  Constant19/1 -> Switch19/3
  Switch65/1 -> Enabled Subsystem65/1(In1)
  Constant4/1 -> Switch4/3
  Constant96/1 -> Switch96/3
  Enabled Subsystem67/1(Out1) -> out64/1, Delay59/1
  Delay75/1 -> Switch92/1
  Delay11/1 -> Switch12/1
  Constant51/1 -> Switch51/3
  Enabled Subsystem11/1(Out1) -> out12/1, Delay11/1
  Switch11/1 -> Enabled Subsystem11/1(In1)
  Constant94/1 -> Switch94/3
  Switch28/1 -> Enabled Subsystem28/1(In1)
  Constant80/1 -> Switch80/3
  Constant74/1 -> Switch74/3
  Switch27/1 -> Enabled Subsystem27/1(In1)
  Enabled Subsystem10/1(Out1) -> out11/1, Delay10/1
  Delay97/1 -> Switch80/1
  Enabled Subsystem/1(Out1) -> out1/1, Delay/1
  Switch95/1 -> Enabled Subsystem95/1(In1)
  Switch99/1 -> Enabled Subsystem99/1(In1)
  Switch12/1 -> Enabled Subsystem12/1(In1)
  Switch19/1 -> Enabled Subsystem19/1(In1)
  Switch36/1 -> Enabled Subsystem36/1(In1)
  Constant87/1 -> Switch87/3
  Delay7/1 -> Switch8/1
  Constant30/1 -> Switch30/3
  Enabled Subsystem50/1(Out1) -> out59/1, Delay55/1
  Switch51/1 -> Enabled Subsystem51/1(In1)
  Constant33/1 -> Switch33/3
  Enabled Subsystem60/1(Out1) -> out76/1, Delay70/1
  Delay28/1 -> Switch39/1
  Enabled Subsystem54/1(Out1) -> out62/1, Delay57/1
  Delay41/1 -> Switch74/1
  Delay3/1 -> Switch4/1
  Constant8/1 -> Switch8/3
  Constant72/1 -> Switch72/3
  Switch61/1 -> Enabled Subsystem61/1(In1)
  Constant18/1 -> Switch18/3
  Delay79/1 -> Switch96/1
  Enabled Subsystem93/1(Out1) -> out84/1, Delay77/1
  Delay88/1 -> Switch88/1
  Constant67/1 -> Switch67/3
  Switch97/1 -> Enabled Subsystem97/1(In1)
  data_in/1 -> Switch/1
  Enabled Subsystem13/1(Out1) -> out14/1, Delay13/1
  Constant82/1 -> Switch82/3
  Constant15/1 -> Switch15/3
  Switch93/1 -> Enabled Subsystem93/1(In1)
  Delay61/1 -> Switch70/1
  Logical Operator/1 -> Switch91/2, Switch90/2, Switch89/2, Switch88/2, Switch87/2, Switch86/2, Switch85/2, Switch84/2, Switch83/2, Switch82/2, Switch99/2, Switch98/2, Switch97/2, Switch96/2, Switch95/2, Switch94/2, Switch93/2, Switch92/2, Switch81/2, Switch80/2, Switch65/2, Switch64/2, Switch62/2, Switch61/2, Switch60/2, Switch59/2, Switch58/2, Switch57/2, Switch56/2, Switch55/2, Switch73/2, Switch72/2, Switch71/2, Switch70/2, Switch69/2, Switch68/2, Switch67/2, Switch66/2, Switch54/2, Switch53/2, Switch51/2, Switch50/2, Switch49/2, Switch48/2, Switch47/2, Switch46/2, Switch45/2, Switch44/2, Switch43/2, Switch42/2, Switch79/2, Switch78/2, Switch77/2, Switch76/2, Switch75/2, Switch74/2, Switch63/2, Switch52/2, Switch41/2, Switch40/2, Switch31/2, Switch30/2, Switch29/2, Switch28/2, Switch27/2, Switch26/2, Switch25/2, Switch24/2, Switch23/2, Switch22/2, Switch39/2, Switch38/2, Switch37/2, Switch36/2, Switch35/2, Switch34/2, Switch33/2, Switch32/2, Switch21/2, Switch20/2, Switch19/2, Switch18/2, Switch17/2, Switch16/2, Switch15/2, Switch14/2, Switch13/2, Switch12/2, Switch11/2, Switch10/2, Switch9/2, Switch8/2, Switch7/2, Switch6/2, Switch5/2, Switch4/2, Switch3/2, Switch2/2, Switch1/2, Switch/2
  Delay85/1 -> Switch85/1
  Switch25/1 -> Enabled Subsystem25/1(In1)
  Enabled Subsystem18/1(Out1) -> out19/1, Delay18/1
  Enabled Subsystem29/1(Out1) -> out38/1, Delay36/1
  Switch80/1 -> Enabled Subsystem80/1(In1)
  Enabled Subsystem12/1(Out1) -> out13/1, Delay12/1
  Enabled Subsystem20/1(Out1) -> out21/1, Delay20/1
  Switch21/1 -> Enabled Subsystem21/1(In1)
  Delay18/1 -> Switch19/1
  Enabled Subsystem34/1(Out1) -> out25/1, Delay24/1
  Enabled Subsystem47/1(Out1) -> out56/1, Delay52/1
  Constant86/1 -> Switch86/3
  Constant35/1 -> Switch35/3
  Delay9/1 -> Switch10/1
  Constant13/1 -> Switch13/3
  Delay93/1 -> Switch40/1
  Enabled Subsystem66/1(Out1) -> out63/1, Delay58/1
  Delay59/1 -> Switch68/1
  Enabled Subsystem57/1(Out1) -> out73/1, Delay67/1
  Switch88/1 -> Enabled Subsystem88/1(In1)
  Constant66/1 -> Switch66/3
  Delay32/1 -> Switch26/1
  Constant88/1 -> Switch88/3
  Enabled Subsystem30/1(Out1) -> out39/1, Delay37/1
  Switch79/1 -> Enabled Subsystem79/1(In1)
  Constant89/1 -> Switch89/3
  Enabled Subsystem61/1(Out1) -> out77/1, Delay71/1
  Delay16/1 -> Switch17/1
  Switch56/1 -> Enabled Subsystem56/1(In1)
  Enabled Subsystem85/1(Out1) -> out94/1, Delay86/1
  Enabled Subsystem64/1(Out1) -> out79/1, Delay73/1
  Delay71/1 -> Switch62/1
  Enabled Subsystem80/1(Out1) -> out81/1, Delay74/1
  Enabled Subsystem71/1(Out1) -> out68/1, Delay63/1
  Enabled Subsystem84/1(Out1) -> out93/1, Delay85/1
  Enabled Subsystem7/1(Out1) -> out8/1, Delay7/1
  Switch75/1 -> Enabled Subsystem75/1(In1)
  Switch18/1 -> Enabled Subsystem18/1(In1)
  Delay38/1 -> Switch41/1
  Constant85/1 -> Switch85/3
  Switch47/1 -> Enabled Subsystem47/1(In1)
  Constant91/1 -> Switch91/3
  Constant26/1 -> Switch26/3
  Delay2/1 -> Switch3/1
  Delay57/1 -> Switch66/1
  Constant20/1 -> Switch20/3
  Delay82/1 -> Switch99/1
  Enabled Subsystem22/1(Out1) -> out31/1, Delay29/1
  Delay70/1 -> Switch61/1
  Delay33/1 -> Switch27/1
  Constant60/1 -> Switch60/3
  Delay95/1 -> Switch53/1
  Constant32/1 -> Switch32/3
  Switch87/1 -> Enabled Subsystem87/1(In1)
  Enabled Subsystem82/1(Out1) -> out91/1, Delay83/1
  Switch92/1 -> Enabled Subsystem92/1(In1)
  Delay13/1 -> Switch14/1
  Delay47/1 -> Switch43/1
  Constant98/1 -> Switch98/3
  Switch81/1 -> Enabled Subsystem81/1(In1)
  Delay96/1 -> Switch55/1
  Delay35/1 -> Switch29/1
  Delay73/1 -> Switch65/1
  Enabled Subsystem96/1(Out1) -> out87/1, Delay80/1
  Enabled Subsystem3/1(Out1) -> out4/1, Delay3/1
  Constant23/1 -> Switch23/3
  Constant90/1 -> Switch90/3
  Enabled Subsystem25/1(Out1) -> out34/1, Delay32/1
  Enabled Subsystem69/1(Out1) -> out66/1, Delay61/1
  Constant78/1 -> Switch78/3
  Constant27/1 -> Switch27/3
  Delay14/1 -> Switch15/1
  Enabled Subsystem4/1(Out1) -> out5/1, Delay4/1
  Constant36/1 -> Switch36/3
  Switch39/1 -> Enabled Subsystem39/1(In1)
  Delay42/1 -> Switch75/1
  Enabled Subsystem14/1(Out1) -> out15/1, Delay14/1
  Enabled Subsystem46/1(Out1) -> out55/1, Delay51/1
  Switch57/1 -> Enabled Subsystem57/1(In1)
  Delay87/1 -> Switch87/1
  Enabled Subsystem37/1(Out1) -> out28/1, Delay27/1
  Constant84/1 -> Switch84/3
  Constant1/1 -> Switch1/3
  Enabled Subsystem73/1(Out1) -> out70/1, Delay96/1
  Switch41/1 -> Enabled Subsystem41/1(In1)
  Delay20/1 -> Switch21/1
  Delay68/1 -> Switch59/1
  Switch98/1 -> Enabled Subsystem98/1(In1)
  Delay43/1 -> Switch76/1
  Constant65/1 -> Switch65/3
  Constant17/1 -> Switch17/3
  Switch60/1 -> Enabled Subsystem60/1(In1)
  Enabled Subsystem62/1(Out1) -> out78/1, Delay72/1
  Constant7/1 -> Switch7/3
  Delay78/1 -> Switch95/1
  Enabled Subsystem91/1(Out1) -> out100/1
  Switch40/1 -> Enabled Subsystem40/1(In1)
  Switch78/1 -> Enabled Subsystem78/1(In1)
  Switch85/1 -> Enabled Subsystem85/1(In1)
  Delay12/1 -> Switch13/1
  Switch86/1 -> Enabled Subsystem86/1(In1)
  Delay84/1 -> Switch84/1
  Constant77/1 -> Switch77/3
  Delay6/1 -> Switch7/1
  Constant42/1 -> Switch42/3
  Delay80/1 -> Switch97/1
  Delay53/1 -> Switch49/1
  Enabled Subsystem28/1(Out1) -> out37/1, Delay35/1
  Enabled Subsystem70/1(Out1) -> out67/1, Delay62/1
  Enabled Subsystem2/1(Out1) -> out3/1, Delay2/1
  Enabled Subsystem94/1(Out1) -> out85/1, Delay78/1
  Constant10/1 -> Switch10/3
  Enabled Subsystem87/1(Out1) -> out96/1, Delay88/1
  enable/1 -> Logical Operator1/1
  Enabled Subsystem23/1(Out1) -> out32/1, Delay30/1
  Delay26/1 -> Switch37/1
  Switch62/1 -> Enabled Subsystem62/1(In1)
  Enabled Subsystem41/1(Out1) -> out42/1, Delay39/1
  Delay83/1 -> Switch83/1
  Delay45/1 -> Switch78/1
  Switch10/1 -> Enabled Subsystem10/1(In1)
  Enabled Subsystem38/1(Out1) -> out29/1, Delay28/1
  Enabled Subsystem92/1(Out1) -> out83/1, Delay76/1
  Delay5/1 -> Switch6/1
  Switch53/1 -> Enabled Subsystem53/1(In1)
  Enabled Subsystem26/1(Out1) -> out35/1, Delay33/1
  Switch48/1 -> Enabled Subsystem48/1(In1)
  Delay55/1 -> Switch51/1
  Delay34/1 -> Switch28/1
  Switch7/1 -> Enabled Subsystem7/1(In1)
  Enabled Subsystem86/1(Out1) -> out95/1, Delay87/1
  Delay10/1 -> Switch11/1
  Enabled Subsystem99/1(Out1) -> out90/1, Delay98/1
  Constant52/1 -> Switch52/3
  Switch96/1 -> Enabled Subsystem96/1(In1)
  Constant44/1 -> Switch44/3
  Delay69/1 -> Switch60/1
  Enabled Subsystem31/1(Out1) -> out40/1, Delay93/1
  Enabled Subsystem79/1(Out1) -> out50/1, Delay94/1
  Switch46/1 -> Enabled Subsystem46/1(In1)
  Delay30/1 -> Switch24/1
  Enabled Subsystem33/1(Out1) -> out24/1, Delay23/1
  Enabled Subsystem9/1(Out1) -> out10/1, Delay9/1
  Enabled Subsystem19/1(Out1) -> out20/1, Delay19/1
  Switch5/1 -> Enabled Subsystem5/1(In1)
  Constant69/1 -> Switch69/3
  Enabled Subsystem42/1(Out1) -> out51/1, Delay47/1
  Delay17/1 -> Switch18/1
  Constant45/1 -> Switch45/3
  Delay46/1 -> Switch79/1
  Enabled Subsystem81/1(Out1) -> out82/1, Delay75/1
  Enabled Subsystem35/1(Out1) -> out26/1, Delay25/1
  Enabled Subsystem24/1(Out1) -> out33/1, Delay31/1
  Delay15/1 -> Switch16/1
  Delay54/1 -> Switch50/1
  Enabled Subsystem83/1(Out1) -> out92/1, Delay84/1
  Constant57/1 -> Switch57/3
  Delay49/1 -> Switch45/1
  Delay74/1 -> Switch81/1
  Delay4/1 -> Switch5/1
  Enabled Subsystem43/1(Out1) -> out52/1, Delay48/1
  Switch67/1 -> Enabled Subsystem67/1(In1)
  Constant5/1 -> Switch5/3
  Switch42/1 -> Enabled Subsystem42/1(In1)
  Constant14/1 -> Switch14/3
  Switch91/1 -> Enabled Subsystem91/1(In1)
  Enabled Subsystem45/1(Out1) -> out54/1, Delay50/1
  Delay63/1 -> Switch72/1
  Delay44/1 -> Switch77/1
  Delay60/1 -> Switch69/1
  Switch50/1 -> Enabled Subsystem50/1(In1)
  Enabled Subsystem21/1(Out1) -> out22/1, Delay21/1
  Delay19/1 -> Switch20/1
  reset/1 -> Logical Operator1/2, Logical Operator/1
  Constant43/1 -> Switch43/3
  Delay40/1 -> Switch63/1
  Enabled Subsystem40/1(Out1) -> out41/1, Delay38/1
  Switch69/1 -> Enabled Subsystem69/1(In1)
  Enabled Subsystem51/1(Out1) -> out60/1, Delay95/1
  Delay91/1 -> Switch91/1
  Constant25/1 -> Switch25/3
  Delay21/1 -> Switch32/1
  Enabled Subsystem95/1(Out1) -> out86/1, Delay79/1
  Enabled Subsystem32/1(Out1) -> out23/1, Delay22/1
  Delay51/1 -> Switch47/1
  Switch20/1 -> Enabled Subsystem20/1(In1)
  Switch84/1 -> Enabled Subsystem84/1(In1)
  Switch9/1 -> Enabled Subsystem9/1(In1)
  Delay62/1 -> Switch71/1
  Enabled Subsystem27/1(Out1) -> out36/1, Delay34/1
  Enabled Subsystem90/1(Out1) -> out99/1, Delay91/1
  Switch54/1 -> Enabled Subsystem54/1(In1)
  Enabled Subsystem98/1(Out1) -> out89/1, Delay82/1
  Delay66/1 -> Switch57/1
  Switch22/1 -> Enabled Subsystem22/1(In1)
  Switch68/1 -> Enabled Subsystem68/1(In1)
  Delay56/1 -> Switch54/1
  Constant95/1 -> Switch95/3
  Switch24/1 -> Enabled Subsystem24/1(In1)
  Enabled Subsystem6/1(Out1) -> out7/1, Delay6/1
  Constant3/1 -> Switch3/3
  Enabled Subsystem89/1(Out1) -> out98/1, Delay90/1
  Switch16/1 -> Enabled Subsystem16/1(In1)
  Switch49/1 -> Enabled Subsystem49/1(In1)
  Enabled Subsystem58/1(Out1) -> out74/1, Delay68/1
  Switch71/1 -> Enabled Subsystem71/1(In1)
  Switch64/1 -> Enabled Subsystem64/1(In1)
  Enabled Subsystem75/1(Out1) -> out46/1, Delay43/1
  Logical Operator1/1 -> Enabled Subsystem/Enable, Enabled Subsystem1/Enable, Enabled Subsystem9/Enable, Enabled Subsystem8/Enable, Enabled Subsystem7/Enable, Enabled Subsystem6/Enable, Enabled Subsystem5/Enable, Enabled Subsystem4/Enable, Enabled Subsystem3/Enable, Enabled Subsystem2/Enable, Enabled Subsystem81/Enable, Enabled Subsystem99/Enable, Enabled Subsystem98/Enable, Enabled Subsystem97/Enable, Enabled Subsystem96/Enable, Enabled Subsystem95/Enable, Enabled Subsystem94/Enable, Enabled Subsystem93/Enable, Enabled Subsystem92/Enable, Enabled Subsystem80/Enable, Enabled Subsystem91/Enable, Enabled Subsystem90/Enable, Enabled Subsystem89/Enable, Enabled Subsystem88/Enable, Enabled Subsystem87/Enable, Enabled Subsystem86/Enable, Enabled Subsystem85/Enable, Enabled Subsystem84/Enable, Enabled Subsystem83/Enable, Enabled Subsystem82/Enable, Enabled Subsystem65/Enable, Enabled Subsystem64/Enable, Enabled Subsystem62/Enable, Enabled Subsystem61/Enable, Enabled Subsystem60/Enable, Enabled Subsystem59/Enable, Enabled Subsystem58/Enable, Enabled Subsystem57/Enable, Enabled Subsystem56/Enable, Enabled Subsystem55/Enable, Enabled Subsystem54/Enable, Enabled Subsystem73/Enable, Enabled Subsystem72/Enable, Enabled Subsystem71/Enable, Enabled Subsystem70/Enable, Enabled Subsystem69/Enable, Enabled Subsystem68/Enable, Enabled Subsystem67/Enable, Enabled Subsystem66/Enable, Enabled Subsystem53/Enable, Enabled Subsystem43/Enable, Enabled Subsystem51/Enable, Enabled Subsystem50/Enable, Enabled Subsystem49/Enable, Enabled Subsystem48/Enable, Enabled Subsystem47/Enable, Enabled Subsystem46/Enable, Enabled Subsystem45/Enable, Enabled Subsystem44/Enable, Enabled Subsystem42/Enable, Enabled Subsystem41/Enable, Enabled Subsystem79/Enable, Enabled Subsystem78/Enable, Enabled Subsystem77/Enable, Enabled Subsystem76/Enable, Enabled Subsystem75/Enable, Enabled Subsystem74/Enable, Enabled Subsystem63/Enable, Enabled Subsystem52/Enable, Enabled Subsystem40/Enable, Enabled Subsystem31/Enable, Enabled Subsystem30/Enable, Enabled Subsystem29/Enable, Enabled Subsystem28/Enable, Enabled Subsystem27/Enable, Enabled Subsystem26/Enable, Enabled Subsystem25/Enable, Enabled Subsystem24/Enable, Enabled Subsystem23/Enable, Enabled Subsystem22/Enable, Enabled Subsystem39/Enable, Enabled Subsystem38/Enable, Enabled Subsystem37/Enable, Enabled Subsystem36/Enable, Enabled Subsystem35/Enable, Enabled Subsystem34/Enable, Enabled Subsystem33/Enable, Enabled Subsystem32/Enable, Enabled Subsystem21/Enable, Enabled Subsystem20/Enable, Enabled Subsystem10/Enable, Enabled Subsystem19/Enable, Enabled Subsystem18/Enable, Enabled Subsystem17/Enable, Enabled Subsystem16/Enable, Enabled Subsystem15/Enable, Enabled Subsystem14/Enable, Enabled Subsystem13/Enable, Enabled Subsystem12/Enable, Enabled Subsystem11/Enable
  Constant16/1 -> Switch16/3
  Delay23/1 -> Switch34/1
  Switch1/1 -> Enabled Subsystem1/1(In1)
  Constant79/1 -> Switch79/3
  Switch/1 -> Enabled Subsystem/1(In1)
  Switch30/1 -> Enabled Subsystem30/1(In1)
  Delay1/1 -> Switch2/1
  Enabled Subsystem15/1(Out1) -> out16/1, Delay15/1
  Enabled Subsystem56/1(Out1) -> out72/1, Delay66/1
  Enabled Subsystem78/1(Out1) -> out49/1, Delay46/1
  Enabled Subsystem68/1(Out1) -> out65/1, Delay60/1
  Constant48/1 -> Switch48/3
  Enabled Subsystem65/1(Out1) -> out80/1, Delay97/1
  Enabled Subsystem88/1(Out1) -> out97/1, Delay89/1
  Switch66/1 -> Enabled Subsystem66/1(In1)
  Enabled Subsystem8/1(Out1) -> out9/1, Delay8/1
  Switch59/1 -> Enabled Subsystem59/1(In1)
  Switch35/1 -> Enabled Subsystem35/1(In1)
  Constant21/1 -> Switch21/3
  Enabled Subsystem74/1(Out1) -> out45/1, Delay42/1
  Enabled Subsystem16/1(Out1) -> out17/1, Delay16/1
  Switch43/1 -> Enabled Subsystem43/1(In1)
  Constant63/1 -> Switch63/3
